simulink model "PIDedited"  (R2016b)
settings: Solver=VariableStepAuto  StartTime=0.0  StopTime=20  RelTol=1e-3
libraries: cstblocks x3
settings Model: Creator=diamond  LastModifiedBy=diamond

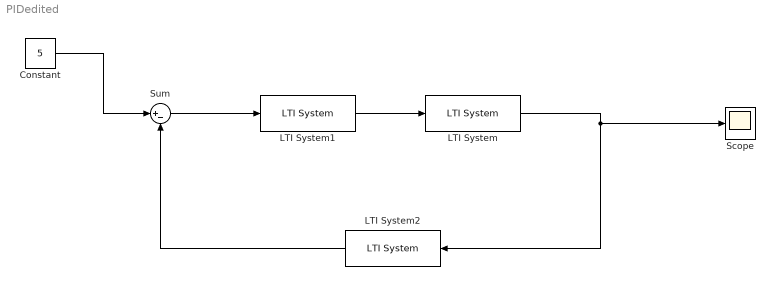
== system PIDedited ==
  Constant : Constant  Value=5
  LTI System : cstblocks/LTI System  sys=tf([10/3],[1,8.16])  IC=[]
  LTI System1 : cstblocks/LTI System  sys=tf([12.44,67.18,90.68],[1,-8.16,0])  IC=[]
  LTI System2 : cstblocks/LTI System  sys=tf([1],[1])  IC=[]
  Scope : Scope
  Sum : Sum  Inputs=|+-
  wires:
  LTI System1/1 -> LTI System/1
  LTI System/1 -> Scope/1, LTI System2/1
  Sum/1 -> LTI System1/1
  LTI System2/1 -> Sum/2
  Constant/1 -> Sum/1
